simulink model "APPL_PaFaultDetection"  (R2018b)
settings: configuration reference "CodeConfig_10_ms" (kept outside this file)
undefined symbols (not defined in the file): CAL_LockErrNoTime_30ms, CAL_ManualSwValid_90s, CAL_MotorHallInvalid_2s, CAL_MotorMaxRunTime_60s, CAL_MotorRelayErr_2s, CAL_MotorStall_750ms, D_DrSoftStopDef_B, D_DrSoftStopDef_F, D_DrSoftStopDef_H, D_DrSoftStopDef_L, D_Relay_DownBackFault, D_Relay_UpFrontFault, D_StallCurrent, enSeatMoveCmd, FALSE, TRUE
libraries: DareLib x91, simulink x2
(part 2 of 4)

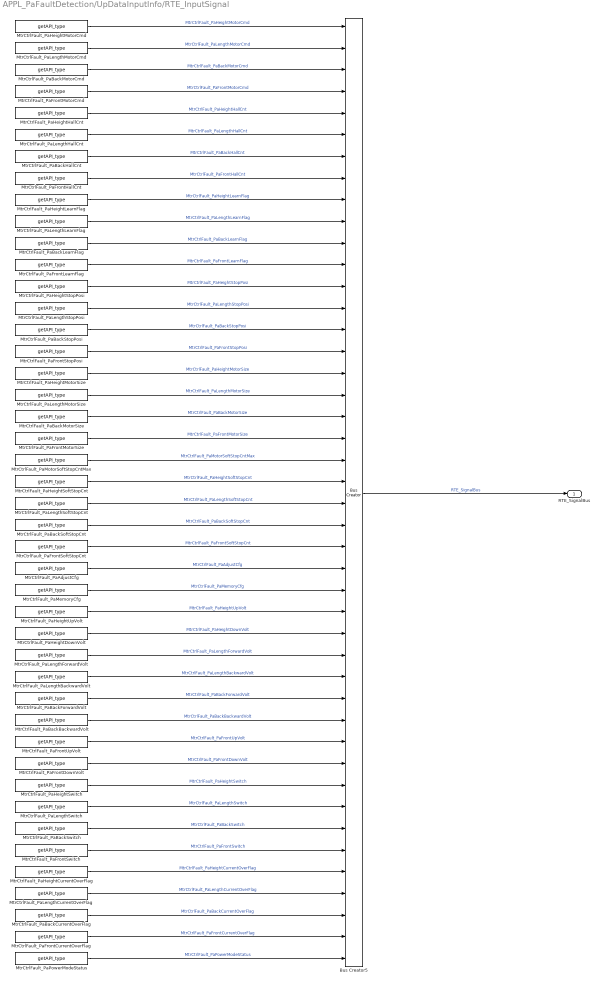
== system APPL_PaFaultDetection/UpDataInputInfo/RTE_InputSignal ==
  Bus Creator5 : BusCreator  Inputs=44
  MtrCtrlFault_PaAdjustCfg : DareLib/Dare/getAPI_type  g_funcname=Srvl_GetMemIndexDataU8  g_param=EN_MemIndex_PaAdjustConfig  g_type=uint8  g_size=-1
      settings: AttributesFormatString=%<g_funcname>  SourceProductName=Dare Library
  MtrCtrlFault_PaBackBackwardVolt : DareLib/Dare/getAPI_type  g_funcname=Ecual_GetPaRelayFlagBackBackward  g_param=""  g_type=uint8  g_size=-1
      settings: AttributesFormatString=%<g_funcname>  SourceProductName=Dare Library
  MtrCtrlFault_PaBackCurrentOverFlag : DareLib/Dare/getAPI_type  g_funcname=Ecual_GetPrBackOverCurrentFlag  g_param=""  g_type=uint8  g_size=-1
      settings: AttributesFormatString=%<g_funcname>  SourceProductName=Dare Library
  MtrCtrlFault_PaBackForwardVolt : DareLib/Dare/getAPI_type  g_funcname=Ecual_GetPaRelayFlagBackForward  g_param=""  g_type=uint8  g_size=-1
      settings: AttributesFormatString=%<g_funcname>  SourceProductName=Dare Library
  MtrCtrlFault_PaBackHallCnt : DareLib/Dare/getAPI_type  g_funcname=Cdd_GetCurrentHallCnt  g_param=EN_PassengerBack  g_type=uint16  g_size=-1
      settings: AttributesFormatString=%<g_funcname>  SourceProductName=Dare Library
  MtrCtrlFault_PaBackLearnFlag : DareLib/Dare/getAPI_type  g_funcname=Cdd_GetMotorLearnFlag  g_param=EN_PassengerBack  g_type=uint8  g_size=-1
      settings: AttributesFormatString=%<g_funcname>  SourceProductName=Dare Library
  MtrCtrlFault_PaBackMotorCmd : DareLib/Dare/getAPI_type  g_funcname=Rte_GetVfb_PaBackMotorCmd  g_param=""  g_type=uint8  g_size=-1
      settings: AttributesFormatString=%<g_funcname>  SourceProductName=Dare Library
  MtrCtrlFault_PaBackMotorSize : DareLib/Dare/getAPI_type  g_funcname=Cdd_GetMotorSize  g_param=EN_PassengerBack  g_type=uint16  g_size=-1
      settings: AttributesFormatString=%<g_funcname>  SourceProductName=Dare Library
  MtrCtrlFault_PaBackSoftStopCnt : DareLib/Dare/getAPI_type  g_funcname=Srvl_GetMemIndexDataU8  g_param=EN_MemIndex_PaBackSoftStopCnt  g_type=uint8  g_size=-1
      settings: AttributesFormatString=%<g_funcname>  SourceProductName=Dare Library
  MtrCtrlFault_PaBackStopPosi : DareLib/Dare/getAPI_type  g_funcname=Cdd_GetMotorHardStop  g_param=EN_PassengerBack  g_type=uint16  g_size=-1
      settings: AttributesFormatString=%<g_funcname>  SourceProductName=Dare Library
  MtrCtrlFault_PaBackSwitch : DareLib/Dare/getAPI_type  g_funcname=Ecual_GetPaBackSwitchCmd  g_param=""  g_type=uint8  g_enum=enSeatMoveCmd  g_size=-1
      settings: AttributesFormatString=%<g_funcname>  SourceProductName=Dare Library
  MtrCtrlFault_PaFrontCurrentOverFlag : DareLib/Dare/getAPI_type  g_funcname=Ecual_GetPrFrontOverCurrentFlag  g_param=""  g_type=uint8  g_size=-1
      settings: AttributesFormatString=%<g_funcname>  SourceProductName=Dare Library
  MtrCtrlFault_PaFrontDownVolt : DareLib/Dare/getAPI_type  g_funcname=Ecual_GetPaRelayFlagFrontDown  g_param=""  g_type=uint8  g_size=-1
      settings: AttributesFormatString=%<g_funcname>  SourceProductName=Dare Library
  MtrCtrlFault_PaFrontHallCnt : DareLib/Dare/getAPI_type  g_funcname=Cdd_GetCurrentHallCnt  g_param=EN_PaResever_2  g_type=uint16  g_size=-1
      settings: AttributesFormatString=%<g_funcname>  SourceProductName=Dare Library
  MtrCtrlFault_PaFrontLearnFlag : DareLib/Dare/getAPI_type  g_funcname=Cdd_GetMotorLearnFlag  g_param=EN_PaResever_2  g_type=uint8  g_size=-1
      settings: AttributesFormatString=%<g_funcname>  SourceProductName=Dare Library
  MtrCtrlFault_PaFrontMotorCmd : DareLib/Dare/getAPI_type  g_funcname=Rte_GetVfb_PaFrontMotorCmd  g_param=""  g_type=uint8  g_size=-1
      settings: AttributesFormatString=%<g_funcname>  SourceProductName=Dare Library
  MtrCtrlFault_PaFrontMotorSize : DareLib/Dare/getAPI_type  g_funcname=Cdd_GetMotorSize  g_param=EN_PaResever_2  g_type=uint16  g_size=-1
      settings: AttributesFormatString=%<g_funcname>  SourceProductName=Dare Library
  MtrCtrlFault_PaFrontSoftStopCnt : DareLib/Dare/getAPI_type  g_funcname=Srvl_GetMemIndexDataU8  g_param=EN_MemIndex_PaFrontSoftStopCnt  g_type=uint8  g_size=-1
      settings: AttributesFormatString=%<g_funcname>  SourceProductName=Dare Library
  MtrCtrlFault_PaFrontStopPosi : DareLib/Dare/getAPI_type  g_funcname=Cdd_GetMotorHardStop  g_param=EN_PaResever_2  g_type=uint16  g_size=-1
      settings: AttributesFormatString=%<g_funcname>  SourceProductName=Dare Library
  MtrCtrlFault_PaFrontSwitch : DareLib/Dare/getAPI_type  g_funcname=Ecual_GetPaFrontSwitchCmd  g_param=""  g_type=uint8  g_enum=enSeatMoveCmd  g_size=-1
      settings: AttributesFormatString=%<g_funcname>  SourceProductName=Dare Library
  MtrCtrlFault_PaFrontUpVolt : DareLib/Dare/getAPI_type  g_funcname=Ecual_GetPaRelayFlagFrontUp  g_param=""  g_type=uint8  g_size=-1
      settings: AttributesFormatString=%<g_funcname>  SourceProductName=Dare Library
  MtrCtrlFault_PaHeightCurrentOverFlag : DareLib/Dare/getAPI_type  g_funcname=Ecual_GetPrHeightOverCurrentFlag  g_param=""  g_type=uint8  g_size=-1
      settings: AttributesFormatString=%<g_funcname>  SourceProductName=Dare Library
  MtrCtrlFault_PaHeightDownVolt : DareLib/Dare/getAPI_type  g_funcname=Ecual_GetPaRelayFlagHeightDN  g_param=""  g_type=uint8  g_size=-1
      settings: AttributesFormatString=%<g_funcname>  SourceProductName=Dare Library
  MtrCtrlFault_PaHeightHallCnt : DareLib/Dare/getAPI_type  g_funcname=Cdd_GetCurrentHallCnt  g_param=EN_PaResever_1  g_type=uint16  g_size=-1
      settings: AttributesFormatString=%<g_funcname>  SourceProductName=Dare Library
  MtrCtrlFault_PaHeightLearnFlag : DareLib/Dare/getAPI_type  g_funcname=Cdd_GetMotorLearnFlag  g_param=EN_PaResever_1  g_type=uint8  g_size=-1
      settings: AttributesFormatString=%<g_funcname>  SourceProductName=Dare Library
  MtrCtrlFault_PaHeightMotorCmd : DareLib/Dare/getAPI_type  g_funcname=Rte_GetVfb_PaHeightMotorCmd  g_param=""  g_type=uint8  g_size=-1
      settings: AttributesFormatString=%<g_funcname>  SourceProductName=Dare Library
  MtrCtrlFault_PaHeightMotorSize : DareLib/Dare/getAPI_type  g_funcname=Cdd_GetMotorSize  g_param=EN_PaResever_1  g_type=uint16  g_size=-1
      settings: AttributesFormatString=%<g_funcname>  SourceProductName=Dare Library
  MtrCtrlFault_PaHeightSoftStopCnt : DareLib/Dare/getAPI_type  g_funcname=Srvl_GetMemIndexDataU8  g_param=EN_MemIndex_PaHeightSoftStopCnt  g_type=uint8  g_size=-1
      settings: AttributesFormatString=%<g_funcname>  SourceProductName=Dare Library
  MtrCtrlFault_PaHeightStopPosi : DareLib/Dare/getAPI_type  g_funcname=Cdd_GetMotorHardStop  g_param=EN_PaResever_1  g_type=uint16  g_size=-1
      settings: AttributesFormatString=%<g_funcname>  SourceProductName=Dare Library
  MtrCtrlFault_PaHeightSwitch : DareLib/Dare/getAPI_type  g_funcname=Ecual_GetPaHeightSwitchCmd  g_param=""  g_type=uint8  g_enum=enSeatMoveCmd  g_size=-1
      settings: AttributesFormatString=%<g_funcname>  SourceProductName=Dare Library
  MtrCtrlFault_PaHeightUpVolt : DareLib/Dare/getAPI_type  g_funcname=Ecual_GetPaRelayFlagHeightUp  g_param=""  g_type=uint8  g_size=-1
      settings: AttributesFormatString=%<g_funcname>  SourceProductName=Dare Library
  MtrCtrlFault_PaLengthBackwardVolt : DareLib/Dare/getAPI_type  g_funcname=Ecual_GetPaRelayFlagLenghtBackward  g_param=""  g_type=uint8  g_size=-1
      settings: AttributesFormatString=%<g_funcname>  SourceProductName=Dare Library
  MtrCtrlFault_PaLengthCurrentOverFlag : DareLib/Dare/getAPI_type  g_funcname=Ecual_GetPrLengthOverCurrentFlag  g_param=""  g_type=uint8  g_size=-1
      settings: AttributesFormatString=%<g_funcname>  SourceProductName=Dare Library
  MtrCtrlFault_PaLengthForwardVolt : DareLib/Dare/getAPI_type  g_funcname=Ecual_GetPaRelayFlagLenghtForward  g_param=""  g_type=uint8  g_size=-1
      settings: AttributesFormatString=%<g_funcname>  SourceProductName=Dare Library
  MtrCtrlFault_PaLengthHallCnt : DareLib/Dare/getAPI_type  g_funcname=Cdd_GetCurrentHallCnt  g_param=EN_PassengerLength  g_type=uint16  g_size=-1
      settings: AttributesFormatString=%<g_funcname>  SourceProductName=Dare Library
  MtrCtrlFault_PaLengthLearnFlag : DareLib/Dare/getAPI_type  g_funcname=Cdd_GetMotorLearnFlag  g_param=EN_PassengerLength  g_type=uint8  g_size=-1
      settings: AttributesFormatString=%<g_funcname>  SourceProductName=Dare Library
  MtrCtrlFault_PaLengthMotorCmd : DareLib/Dare/getAPI_type  g_funcname=Rte_GetVfb_PaLengthMotorCmd  g_param=""  g_type=uint8  g_size=-1
      settings: AttributesFormatString=%<g_funcname>  SourceProductName=Dare Library
  MtrCtrlFault_PaLengthMotorSize : DareLib/Dare/getAPI_type  g_funcname=Cdd_GetMotorSize  g_param=EN_PassengerLength  g_type=uint16  g_size=-1
      settings: AttributesFormatString=%<g_funcname>  SourceProductName=Dare Library
  MtrCtrlFault_PaLengthSoftStopCnt : DareLib/Dare/getAPI_type  g_funcname=Srvl_GetMemIndexDataU8  g_param=EN_MemIndex_PaLengthSoftStopCnt  g_type=uint8  g_size=-1
      settings: AttributesFormatString=%<g_funcname>  SourceProductName=Dare Library
  MtrCtrlFault_PaLengthStopPosi : DareLib/Dare/getAPI_type  g_funcname=Cdd_GetMotorHardStop  g_param=EN_PassengerLength  g_type=uint16  g_size=-1
      settings: AttributesFormatString=%<g_funcname>  SourceProductName=Dare Library
  MtrCtrlFault_PaLengthSwitch : DareLib/Dare/getAPI_type  g_funcname=Ecual_GetPaLengthSwitchCmd  g_param=""  g_type=uint8  g_enum=enSeatMoveCmd  g_size=-1
      settings: AttributesFormatString=%<g_funcname>  SourceProductName=Dare Library
  MtrCtrlFault_PaMemoryCfg : DareLib/Dare/getAPI_type  g_funcname=Srvl_GetMemIndexDataU8  g_param=EN_MemIndex_PaMemoryConfig  g_type=uint8  g_size=-1
      settings: AttributesFormatString=%<g_funcname>  SourceProductName=Dare Library
  MtrCtrlFault_PaMotorSoftStopCntMax : DareLib/Dare/getAPI_type  g_funcname=Srvl_GetMemIndexDataU8  g_param=EN_MemIndex_MotorSoftStopCntMax  g_type=uint8  g_size=-1
      settings: AttributesFormatString=%<g_funcname>  SourceProductName=Dare Library
  MtrCtrlFault_PaPowerModeStatus : DareLib/Dare/getAPI_type  g_funcname=Rte_GetVfb_PowerMode  g_param=""  g_type=uint8  g_enum=enIgnSts  g_size=-1
      settings: AttributesFormatString=%<g_funcname>  SourceProductName=Dare Library
  RTE_SignalBus : Outport
  wires:
  Bus Creator5/1 -> RTE_SignalBus/1  "RTE_SignalBus"
  MtrCtrlFault_PaHeightMotorCmd/1 -> Bus Creator5/1  "MtrCtrlFault_PaHeightMotorCmd"
  MtrCtrlFault_PaLengthMotorCmd/1 -> Bus Creator5/2  "MtrCtrlFault_PaLengthMotorCmd"
  MtrCtrlFault_PaBackMotorCmd/1 -> Bus Creator5/3  "MtrCtrlFault_PaBackMotorCmd"
  MtrCtrlFault_PaFrontMotorCmd/1 -> Bus Creator5/4  "MtrCtrlFault_PaFrontMotorCmd"
  MtrCtrlFault_PaHeightHallCnt/1 -> Bus Creator5/5  "MtrCtrlFault_PaHeightHallCnt"
  MtrCtrlFault_PaLengthHallCnt/1 -> Bus Creator5/6  "MtrCtrlFault_PaLengthHallCnt"
  MtrCtrlFault_PaBackHallCnt/1 -> Bus Creator5/7  "MtrCtrlFault_PaBackHallCnt"
  MtrCtrlFault_PaFrontHallCnt/1 -> Bus Creator5/8  "MtrCtrlFault_PaFrontHallCnt"
  MtrCtrlFault_PaHeightLearnFlag/1 -> Bus Creator5/9  "MtrCtrlFault_PaHeightLearnFlag"
  MtrCtrlFault_PaLengthLearnFlag/1 -> Bus Creator5/10  "MtrCtrlFault_PaLengthLearnFlag"
  MtrCtrlFault_PaBackLearnFlag/1 -> Bus Creator5/11  "MtrCtrlFault_PaBackLearnFlag"
  MtrCtrlFault_PaFrontLearnFlag/1 -> Bus Creator5/12  "MtrCtrlFault_PaFrontLearnFlag"
  MtrCtrlFault_PaHeightStopPosi/1 -> Bus Creator5/13  "MtrCtrlFault_PaHeightStopPosi"
  MtrCtrlFault_PaLengthStopPosi/1 -> Bus Creator5/14  "MtrCtrlFault_PaLengthStopPosi"
  MtrCtrlFault_PaBackStopPosi/1 -> Bus Creator5/15  "MtrCtrlFault_PaBackStopPosi"
  MtrCtrlFault_PaFrontStopPosi/1 -> Bus Creator5/16  "MtrCtrlFault_PaFrontStopPosi"
  MtrCtrlFault_PaHeightMotorSize/1 -> Bus Creator5/17  "MtrCtrlFault_PaHeightMotorSize"
  MtrCtrlFault_PaLengthMotorSize/1 -> Bus Creator5/18  "MtrCtrlFault_PaLengthMotorSize"
  MtrCtrlFault_PaBackMotorSize/1 -> Bus Creator5/19  "MtrCtrlFault_PaBackMotorSize"
  MtrCtrlFault_PaFrontMotorSize/1 -> Bus Creator5/20  "MtrCtrlFault_PaFrontMotorSize"
  MtrCtrlFault_PaMotorSoftStopCntMax/1 -> Bus Creator5/21  "MtrCtrlFault_PaMotorSoftStopCntMax"
  MtrCtrlFault_PaHeightSoftStopCnt/1 -> Bus Creator5/22  "MtrCtrlFault_PaHeightSoftStopCnt"
  MtrCtrlFault_PaLengthSoftStopCnt/1 -> Bus Creator5/23  "MtrCtrlFault_PaLengthSoftStopCnt"
  MtrCtrlFault_PaBackSoftStopCnt/1 -> Bus Creator5/24  "MtrCtrlFault_PaBackSoftStopCnt"
  MtrCtrlFault_PaFrontSoftStopCnt/1 -> Bus Creator5/25  "MtrCtrlFault_PaFrontSoftStopCnt"
  MtrCtrlFault_PaAdjustCfg/1 -> Bus Creator5/26  "MtrCtrlFault_PaAdjustCfg"
  MtrCtrlFault_PaMemoryCfg/1 -> Bus Creator5/27  "MtrCtrlFault_PaMemoryCfg"
  MtrCtrlFault_PaHeightUpVolt/1 -> Bus Creator5/28  "MtrCtrlFault_PaHeightUpVolt"
  MtrCtrlFault_PaHeightDownVolt/1 -> Bus Creator5/29  "MtrCtrlFault_PaHeightDownVolt"
  MtrCtrlFault_PaLengthForwardVolt/1 -> Bus Creator5/30  "MtrCtrlFault_PaLengthForwardVolt"
  MtrCtrlFault_PaLengthBackwardVolt/1 -> Bus Creator5/31  "MtrCtrlFault_PaLengthBackwardVolt"
  MtrCtrlFault_PaBackForwardVolt/1 -> Bus Creator5/32  "MtrCtrlFault_PaBackForwardVolt"
  MtrCtrlFault_PaBackBackwardVolt/1 -> Bus Creator5/33  "MtrCtrlFault_PaBackBackwardVolt"
  MtrCtrlFault_PaFrontUpVolt/1 -> Bus Creator5/34  "MtrCtrlFault_PaFrontUpVolt"
  MtrCtrlFault_PaFrontDownVolt/1 -> Bus Creator5/35  "MtrCtrlFault_PaFrontDownVolt"
  MtrCtrlFault_PaHeightSwitch/1 -> Bus Creator5/36  "MtrCtrlFault_PaHeightSwitch"
  MtrCtrlFault_PaLengthSwitch/1 -> Bus Creator5/37  "MtrCtrlFault_PaLengthSwitch"
  MtrCtrlFault_PaBackSwitch/1 -> Bus Creator5/38  "MtrCtrlFault_PaBackSwitch"
  MtrCtrlFault_PaFrontSwitch/1 -> Bus Creator5/39  "MtrCtrlFault_PaFrontSwitch"
  MtrCtrlFault_PaHeightCurrentOverFlag/1 -> Bus Creator5/40  "MtrCtrlFault_PaHeightCurrentOverFlag"
  MtrCtrlFault_PaLengthCurrentOverFlag/1 -> Bus Creator5/41  "MtrCtrlFault_PaLengthCurrentOverFlag"
  MtrCtrlFault_PaBackCurrentOverFlag/1 -> Bus Creator5/42  "MtrCtrlFault_PaBackCurrentOverFlag"
  MtrCtrlFault_PaFrontCurrentOverFlag/1 -> Bus Creator5/43  "MtrCtrlFault_PaFrontCurrentOverFlag"
  MtrCtrlFault_PaPowerModeStatus/1 -> Bus Creator5/44  "MtrCtrlFault_PaPowerModeStatus"

== system APPL_PaFaultDetection/LogicCtrl/AdheAndEffec/SwitchErrorDetection/GetCurMsTs ==
  f : TriggerPort  TriggerType=function-call  VariantControl=(inherit)
      settings: CopyFcn=Stateflow.SLINSF.SimulinkMan.removeBlockPreDeleteFcn  PreDeleteFcn=Stateflow.SLINSF.SimulinkMan.unsafePredeleteFcn
  DrAdj_LenAdjSize : DareLib/Dare/getAPI_type  g_funcname=D_HAL_GET_CUR_MS_TS  g_param=""  g_type=uint32  g_size=-1
      settings: SourceProductName=Dare Library
  Ts : Outport
  wires:
  DrAdj_LenAdjSize/1 -> Ts/1  "DrAdj_CurMsTs"

== system APPL_PaFaultDetection/LogicCtrl/AdheAndEffec/SwitchErrorDetection/GetDefTime ==
  DefTs : Inport
  Ts : Inport  Port=2
  f : TriggerPort  TriggerType=function-call  VariantControl=(inherit)
      settings: CopyFcn=Stateflow.SLINSF.SimulinkMan.removeBlockPreDeleteFcn  PreDeleteFcn=Stateflow.SLINSF.SimulinkMan.unsafePredeleteFcn
  Chart : Stateflow chart  TreatAsAtomicUnit=on
  OutTs : Outport
  wires:
  DefTs/1 -> Chart/1(DefTs)
  Ts/1 -> Chart/2(Ts)
  Chart/1(OutTs) -> OutTs/1

== system APPL_PaFaultDetection/LogicCtrl/AdheAndEffec/SwitchErrorDetection/TimeDiffTs ==
  lastTs : Inport
  Ts : Inport  Port=2
  f : TriggerPort  TriggerType=function-call  VariantControl=(inherit)
      settings: CopyFcn=Stateflow.SLINSF.SimulinkMan.removeBlockPreDeleteFcn  PreDeleteFcn=Stateflow.SLINSF.SimulinkMan.unsafePredeleteFcn
  Chart : Stateflow chart  TreatAsAtomicUnit=on
  OutTs : Outport
  wires:
  lastTs/1 -> Chart/1(lastTs)
  Ts/1 -> Chart/2(Ts)
  Chart/1(OutTs) -> OutTs/1

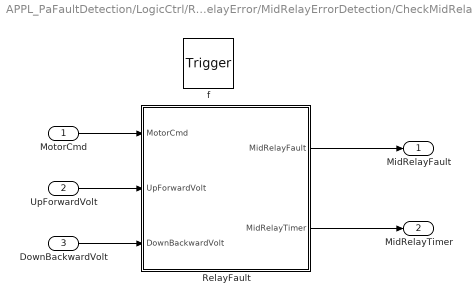
== system APPL_PaFaultDetection/LogicCtrl/RelayError/MidRelayErrorDetection/CheckMidRelayFault ==
  MotorCmd : Inport  OutDataTypeStr=uint8  PortDimensions=1
  UpForwardVolt : Inport  Port=2  OutDataTypeStr=uint8  PortDimensions=1
  DownBackwardVolt : Inport  Port=3  OutDataTypeStr=uint8  PortDimensions=1
  f : TriggerPort  TriggerType=function-call  VariantControl=(inherit)
      settings: CopyFcn=Stateflow.SLINSF.SimulinkMan.removeBlockPreDeleteFcn  PreDeleteFcn=Stateflow.SLINSF.SimulinkMan.unsafePredeleteFcn
  RelayFault : Stateflow chart  TreatAsAtomicUnit=on
  MidRelayFault : Outport  OutDataTypeStr=uint8
  MidRelayTimer : Outport  Port=2  OutDataTypeStr=uint8
  wires:
  MotorCmd/1 -> RelayFault/1(MotorCmd)
  UpForwardVolt/1 -> RelayFault/2(UpForwardVolt)
  DownBackwardVolt/1 -> RelayFault/3(DownBackwardVolt)
  RelayFault/1(MidRelayFault) -> MidRelayFault/1
  RelayFault/2(MidRelayTimer) -> MidRelayTimer/1

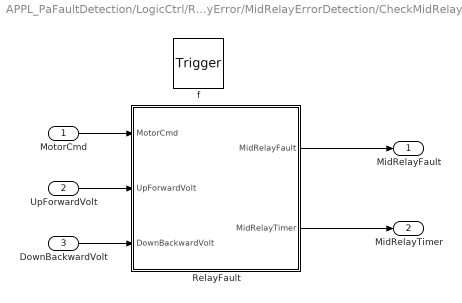
== system APPL_PaFaultDetection/LogicCtrl/RelayError/MidRelayErrorDetection/CheckMidRelayFault1 ==
  MotorCmd : Inport  OutDataTypeStr=uint8  PortDimensions=1
  UpForwardVolt : Inport  Port=2  OutDataTypeStr=uint8  PortDimensions=1
  DownBackwardVolt : Inport  Port=3  OutDataTypeStr=uint8  PortDimensions=1
  f : TriggerPort  TriggerType=function-call  VariantControl=(inherit)
      settings: CopyFcn=Stateflow.SLINSF.SimulinkMan.removeBlockPreDeleteFcn  PreDeleteFcn=Stateflow.SLINSF.SimulinkMan.unsafePredeleteFcn
  RelayFault : Stateflow chart  TreatAsAtomicUnit=on
  MidRelayFault : Outport  OutDataTypeStr=uint8
  MidRelayTimer : Outport  Port=2  OutDataTypeStr=uint8
  wires:
  MotorCmd/1 -> RelayFault/1(MotorCmd)
  UpForwardVolt/1 -> RelayFault/2(UpForwardVolt)
  DownBackwardVolt/1 -> RelayFault/3(DownBackwardVolt)
  RelayFault/1(MidRelayFault) -> MidRelayFault/1
  RelayFault/2(MidRelayTimer) -> MidRelayTimer/1

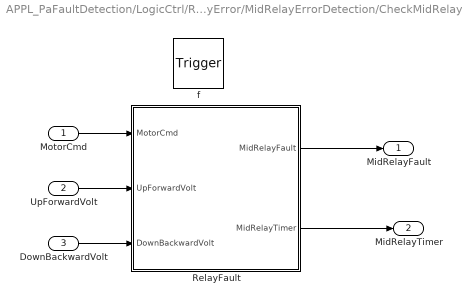
== system APPL_PaFaultDetection/LogicCtrl/RelayError/MidRelayErrorDetection/CheckMidRelayFault2 ==
  MotorCmd : Inport  OutDataTypeStr=uint8  PortDimensions=1
  UpForwardVolt : Inport  Port=2  OutDataTypeStr=uint8  PortDimensions=1
  DownBackwardVolt : Inport  Port=3  OutDataTypeStr=uint8  PortDimensions=1
  f : TriggerPort  TriggerType=function-call  VariantControl=(inherit)
      settings: CopyFcn=Stateflow.SLINSF.SimulinkMan.removeBlockPreDeleteFcn  PreDeleteFcn=Stateflow.SLINSF.SimulinkMan.unsafePredeleteFcn
  RelayFault : Stateflow chart  TreatAsAtomicUnit=on
  MidRelayFault : Outport  OutDataTypeStr=uint8
  MidRelayTimer : Outport  Port=2  OutDataTypeStr=uint8
  wires:
  MotorCmd/1 -> RelayFault/1(MotorCmd)
  UpForwardVolt/1 -> RelayFault/2(UpForwardVolt)
  DownBackwardVolt/1 -> RelayFault/3(DownBackwardVolt)
  RelayFault/1(MidRelayFault) -> MidRelayFault/1
  RelayFault/2(MidRelayTimer) -> MidRelayTimer/1

== system APPL_PaFaultDetection/LogicCtrl/RelayError/MidRelayErrorDetection/CheckMidRelayFault3 ==
  MotorCmd : Inport  OutDataTypeStr=uint8  PortDimensions=1
  UpForwardVolt : Inport  Port=2  OutDataTypeStr=uint8  PortDimensions=1
  DownBackwardVolt : Inport  Port=3  OutDataTypeStr=uint8  PortDimensions=1
  f : TriggerPort  TriggerType=function-call  VariantControl=(inherit)
      settings: CopyFcn=Stateflow.SLINSF.SimulinkMan.removeBlockPreDeleteFcn  PreDeleteFcn=Stateflow.SLINSF.SimulinkMan.unsafePredeleteFcn
  RelayFault : Stateflow chart  TreatAsAtomicUnit=on
  MidRelayFault : Outport  OutDataTypeStr=uint8
  MidRelayTimer : Outport  Port=2  OutDataTypeStr=uint8
  wires:
  MotorCmd/1 -> RelayFault/1(MotorCmd)
  UpForwardVolt/1 -> RelayFault/2(UpForwardVolt)
  DownBackwardVolt/1 -> RelayFault/3(DownBackwardVolt)
  RelayFault/1(MidRelayFault) -> MidRelayFault/1
  RelayFault/2(MidRelayTimer) -> MidRelayTimer/1

== system APPL_PaFaultDetection/LogicCtrl/SoftStopPoint/SoftStopPointDetection/DrAdj_SetBackSoftStopCnt ==
  Cnt : Inport
  f : TriggerPort  TriggerType=function-call  VariantControl=(inherit)
      settings: CopyFcn=Stateflow.SLINSF.SimulinkMan.removeBlockPreDeleteFcn  PreDeleteFcn=Stateflow.SLINSF.SimulinkMan.unsafePredeleteFcn
  DriverFrontMoveType12 : DareLib/Dare/setAPI_type  g_funcname=Srvl_SetMemIndexDataU8  g_param=EN_MemIndex_PaBackSoftStopCnt  g_type=uint8  g_size=-1
      settings: AttributesFormatString=%<g_funcname>  SourceProductName=Dare Library
  wires:
  Cnt/1 -> DriverFrontMoveType12/1

== system APPL_PaFaultDetection/LogicCtrl/SoftStopPoint/SoftStopPointDetection/DrAdj_SetFrontSoftStopCnt ==
  Cnt : Inport
  f : TriggerPort  TriggerType=function-call  VariantControl=(inherit)
      settings: CopyFcn=Stateflow.SLINSF.SimulinkMan.removeBlockPreDeleteFcn  PreDeleteFcn=Stateflow.SLINSF.SimulinkMan.unsafePredeleteFcn
  DriverFrontMoveType12 : DareLib/Dare/setAPI_type  g_funcname=Srvl_SetMemIndexDataU8  g_param=EN_MemIndex_PaFrontSoftStopCnt  g_type=uint8  g_size=-1
      settings: AttributesFormatString=%<g_funcname>  SourceProductName=Dare Library
  wires:
  Cnt/1 -> DriverFrontMoveType12/1

== system APPL_PaFaultDetection/LogicCtrl/SoftStopPoint/SoftStopPointDetection/DrAdj_SetHeightSoftStopCnt ==
  Cnt : Inport
  f : TriggerPort  TriggerType=function-call  VariantControl=(inherit)
      settings: CopyFcn=Stateflow.SLINSF.SimulinkMan.removeBlockPreDeleteFcn  PreDeleteFcn=Stateflow.SLINSF.SimulinkMan.unsafePredeleteFcn
  DriverFrontMoveType12 : DareLib/Dare/setAPI_type  g_funcname=Srvl_SetMemIndexDataU8  g_param=EN_MemIndex_PaHeightSoftStopCnt  g_type=uint8  g_size=-1
      settings: AttributesFormatString=%<g_funcname>  SourceProductName=Dare Library
  wires:
  Cnt/1 -> DriverFrontMoveType12/1

== system APPL_PaFaultDetection/LogicCtrl/SoftStopPoint/SoftStopPointDetection/DrAdj_SetLengthSoftStopCnt ==
  Cnt : Inport
  f : TriggerPort  TriggerType=function-call  VariantControl=(inherit)
      settings: CopyFcn=Stateflow.SLINSF.SimulinkMan.removeBlockPreDeleteFcn  PreDeleteFcn=Stateflow.SLINSF.SimulinkMan.unsafePredeleteFcn
  DriverFrontMoveType12 : DareLib/Dare/setAPI_type  g_funcname=Srvl_SetMemIndexDataU8  g_param=EN_MemIndex_PaLengthSoftStopCnt  g_type=uint8  g_size=-1
      settings: AttributesFormatString=%<g_funcname>  SourceProductName=Dare Library
  wires:
  Cnt/1 -> DriverFrontMoveType12/1

== stateflow chart APPL_PaFaultDetection/LogicCtrl/SwitchErrDeal/ SWProcess  ==
  settings: description=硬线开关信号处理 SWProcess
  state DSM_SWAdjust
    state HeightSWProcess [parallel] [commented out]
      state Enable [commented out]
        en:
        CurrentHeightSwCmd =DrMtr_HeightSwitchCmd;
        du:
        CurrentHeightSwCmd =DrMtr_HeightSwitchCmd;
      state Disable [commented out]
        en:
        CurrentHeightSwCmd = FALSE;
      (default) -> DSM_SWAdjust.HeightSWProcess.Disable [commented out]
      DSM_SWAdjust.HeightSWProcess.Disable -> DSM_SWAdjust.HeightSWProcess.Enable [commented out] : /* 高度本地开关命令故障处理 */
          | [DrMtr_HeightSwitchCmd !=FALSE ...
          | &&FALSE == DrMtr_HeightSwitchAdheErr ...
          | && FALSE ==DrMtr_HeightRelayAdhesionErr ...
          | &&FALSE == DrMtr_HeightStallErr]
      DSM_SWAdjust.HeightSWProcess.Enable -> DSM_SWAdjust.HeightSWProcess.Disable [commented out] : [DrMtr_HeightSwitchCmd ==FALSE ...
          | || FALSE != DrMtr_HeightSwitchAdheErr ...
          | || TRUE == DrMtr_HeightRelayAdhesionErr ...
          | || TRUE == DrMtr_HeightStallErr]
    state LengthSWProcess [parallel]
      settings: executionOrder=1
      state Enable
        en:
        CurrentLengthSwCmd =DrMtr_LengthSwitchCmd;
        du:
        CurrentLengthSwCmd =DrMtr_LengthSwitchCmd;
      state Disable
        en:
        CurrentLengthSwCmd = FALSE;
      (default) -> DSM_SWAdjust.LengthSWProcess.Disable
      DSM_SWAdjust.LengthSWProcess.Disable -> DSM_SWAdjust.LengthSWProcess.Enable : /* 纵向本地开关命令故障处理 */
          | [DrMtr_LengthSwitchCmd !=FALSE ...
          | &&FALSE == DrMtr_LengthSwitchAdheErr...
          | && FALSE ==DrMtr_LengthRelayAdhesionErr ...
          | &&FALSE == DrMtr_LengthStallErr]
      DSM_SWAdjust.LengthSWProcess.Enable -> DSM_SWAdjust.LengthSWProcess.Disable : [DrMtr_LengthSwitchCmd ==FALSE ...
          | || FALSE !=  DrMtr_LengthSwitchAdheErr...
          | || TRUE == DrMtr_LengthRelayAdhesionErr ...
          | || TRUE == DrMtr_LengthStallErr]
    state BackSWProcess [parallel]
      settings: executionOrder=2
      state Enable
        en:
        CurrentBackSwCmd =DrMtr_BackSwitchCmd;
        du:
        CurrentBackSwCmd =DrMtr_BackSwitchCmd;
      state Disable
        en:
        CurrentBackSwCmd = FALSE;
      (default) -> DSM_SWAdjust.BackSWProcess.Disable
      DSM_SWAdjust.BackSWProcess.Disable -> DSM_SWAdjust.BackSWProcess.Enable : /* 靠背本地开关命令故障处理 */
          | [DrMtr_BackSwitchCmd !=FALSE ...
          | &&FALSE == DrMtr_BackRelayAdhesionErr ...
          | &&FALSE == DrMtr_BackSwitchAdheErr...
          | &&FALSE == DrMtr_BackStallErr]
      DSM_SWAdjust.BackSWProcess.Enable -> DSM_SWAdjust.BackSWProcess.Disable : [DrMtr_BackSwitchCmd ==FALSE ...
          | || FALSE != DrMtr_BackRelayAdhesionErr ...
          | || TRUE == DrMtr_BackSwitchAdheErr...
          | || TRUE == DrMtr_BackStallErr]
    state FrontSWProcess [parallel] [commented out]
      state Enable [commented out]
        en:
        CurrentFrontSwCmd =DrMtr_FrontSwitchCmd;
        du:
        CurrentFrontSwCmd =DrMtr_FrontSwitchCmd;
      state Disable [commented out]
        en:
        CurrentFrontSwCmd = FALSE;
      (default) -> DSM_SWAdjust.FrontSWProcess.Disable [commented out]
      DSM_SWAdjust.FrontSWProcess.Disable -> DSM_SWAdjust.FrontSWProcess.Enable [commented out] : /* 腿托本地开关命令故障处理 && 配置字满足*/
          | [DrMtr_FrontSwitchCmd !=FALSE ...
          | && FALSE == DrMtr_FrontSwitchAdheErr...
          | && FALSE ==DrMtr_FrontRelayAdhesionErr ...
          | && FALSE == DrMtr_FrontStallErr ...
          | && EN_DrTwelveWayMotor == MtrCtrlFault_DrAdjustCfg]
      DSM_SWAdjust.FrontSWProcess.Enable -> DSM_SWAdjust.FrontSWProcess.Disable [commented out] : [DrMtr_FrontSwitchCmd ==FALSE ...
          | || FALSE !=  DrMtr_FrontSwitchAdheErr...
          | || TRUE == DrMtr_FrontRelayAdhesionErr ...
          | || TRUE == DrMtr_FrontStallErr...
          | || EN_DrTwelveWayMotor != MtrCtrlFault_DrAdjustCfg]
  state Init
    en:
    CurrentHeightSwCmd = FALSE;
    CurrentLengthSwCmd = FALSE;
    CurrentBackSwCmd = FALSE;
    CurrentFrontSwCmd = FALSE;
  (default) -> Init
  Init -> DSM_SWAdjust : /* 非CRANK档位 且非不可调节配置 */
      | [eCrank != MtrCtrlFault_PowerModeStatus ...
      | && TRUE == MtrCtrlFault_DrAdjustCfg]
  DSM_SWAdjust -> Init : /* crank档 或 不可调节配置 */
      | [eCrank == MtrCtrlFault_PowerModeStatus ...
      | || TRUE != MtrCtrlFault_DrAdjustCfg]
  data: CurrentHeightSwCmd output Enum: enSeatMoveCmd; CurrentLengthSwCmd output Enum: enSeatMoveCmd; CurrentBackSwCmd output Enum: enSeatMoveCmd; DrMtr_HeightSwitchCmd input; DrMtr_LengthSwitchCmd input; DrMtr_BackSwitchCmd input; DrMtr_FrontSwitchCmd input; DrMtr_HeightRelayAdhesionErr input; DrMtr_LengthRelayAdhesionErr input; DrMtr_BackRelayAdhesionErr input; DrMtr_FrontRelayAdhesionErr input; DrMtr_HeightSwitchAdheErr input; DrMtr_LengthSwitchAdheErr input; DrMtr_BackSwitchAdheErr input; DrMtr_FrontSwitchAdheErr input; CurrentFrontSwCmd output Enum: enSeatMoveCmd; FALSE parameter; TRUE parameter; DrMtr_HeightStallErr input; DrMtr_LengthStallErr input; DrMtr_BackStallErr input; DrMtr_FrontStallErr input; MtrCtrlFault_DrAdjustCfg input; MtrCtrlFault_PowerModeStatus input

== stateflow chart APPL_PaFaultDetection/LogicCtrl/RelayError/MidRelayErrorDetection ==
  state [MidRelayFault,MidRelayTimer]  = CheckMidRelayFault(MotorCmd,UpForwardVolt,DownBackwardVolt) [function]
  state [MidRelayFault,MidRelayTimer] = CheckMidRelayFault1(MotorCmd,UpForwardVolt,DownBackwardVolt) [function]
  state [MidRelayFault,MidRelayTimer]  = CheckMidRelayFault2(MotorCmd,UpForwardVolt,DownBackwardVolt) [function]
  state [MidRelayFault,MidRelayTimer]  = CheckMidRelayFault3(MotorCmd,UpForwardVolt,DownBackwardVolt) [function]
  state MidRelayError [parallel]
    settings: executionOrder=1
    (default) -> (junction 66)
    MidRelayError -> (junction 66)
    (junction 66) -> (junction 68) : {/*[HeightMidRelayFault, HeightMidRelayTimer] = CheckMidRelayFault(MtrCtrlFault_HeightMotorCmd,MtrCtrlFault_HeightUpVolt,MtrCtrlFault_HeightDownVolt);*/
        | [LengthMidRelayFault, LengthMidRelayTimer] = CheckMidRelayFault1(MtrCtrlFault_LengthMotorCmd,MtrCtrlFault_LengthForwardVolt,MtrCtrlFault_LengthBackwardVolt);
        | [BackMidRelayFault, BackMidRelayTimer] = CheckMidRelayFault2(MtrCtrlFault_BackMotorCmd,MtrCtrlFault_BackForwardVolt,MtrCtrlFault_BackBackwardVolt);
        | /*[FrontMidRelayFault, FrontMidRelayTimer] = CheckMidRelayFault3(MtrCtrlFault_FrontMotorCmd,MtrCtrlFault_FrontUpVolt,MtrCtrlFault_FrontDownVolt);*/}
  note: 继电器粘连故障检测
  data: MotorCmd function_input uint8 size=1; UpForwardVolt function_input uint8 size=1; DownBackwardVolt function_input uint8 size=1; MidRelayFault function_output uint8; MidRelayTimer function_output uint8; MotorCmd function_input uint8 size=1; UpForwardVolt function_input uint8 size=1; DownBackwardVolt function_input uint8 size=1; MidRelayFault function_output uint8; MidRelayTimer function_output uint8; MotorCmd function_input uint8 size=1; UpForwardVolt function_input uint8 size=1; DownBackwardVolt function_input uint8 size=1; MidRelayFault function_output uint8; MidRelayTimer function_output uint8; MotorCmd function_input uint8 size=1; UpForwardVolt function_input uint8 size=1; DownBackwardVolt function_input uint8 size=1; MidRelayFault function_output uint8; MidRelayTimer function_output uint8; MtrCtrlFault_HeightUpVolt input uint8; MtrCtrlFault_HeightDownVolt input uint8; MtrCtrlFault_LengthForwardVolt input uint8; MtrCtrlFault_LengthBackwardVolt input uint8; MtrCtrlFault_BackForwardVolt input uint8; MtrCtrlFault_BackBackwardVolt input uint8; MtrCtrlFault_FrontUpVolt input uint8; MtrCtrlFault_FrontDownVolt input uint8; MtrCtrlFault_HeightMotorCmd input uint8; MtrCtrlFault_LengthMotorCmd input uint8; MtrCtrlFault_BackMotorCmd input uint8; MtrCtrlFault_FrontMotorCmd input uint8; HeightMidRelayFault output uint8; LengthMidRelayFault output uint8; BackMidRelayFault output uint8; FrontMidRelayFault output uint8; LengthMidRelayTimer local double; BackMidRelayTimer local double; FrontMidRelayTimer local double; HeightMidRelayTimer local double

== stateflow chart APPL_PaFaultDetection/LogicCtrl/RelayError/MidRelayErrorDetection/CheckMidRelayFault/RelayFault ==
  state Judge
    ex:
    MidRelayTimer = 0;
    (default) -> (junction 8)
    Judge -> (junction 8) [order 1]
    (junction 8) -> (junction 10) [order 1] : [CAL_MotorRelayErr_2s <= MidRelayTimer]
    (junction 8) -> (junction 14) [order 2] : {MidRelayTimer ++;}
    (junction 10) -> (junction 12) : {MidRelayTimer = CAL_MotorRelayErr_2s;}
    (junction 12) -> (junction 16) [order 1] : [enSeatMoveCmd.EN_UP_FORWARD != MotorCmd ...
        | && FALSE != UpForwardVolt]
    (junction 12) -> (junction 20) [order 2]
    (junction 16) -> (junction 18) : {MidRelayFault = D_Relay_UpFrontFault;}
    (junction 20) -> (junction 23) [order 1] : [enSeatMoveCmd.EN_DN_BACKWARD != MotorCmd ...
        | && FALSE != DownBackwardVolt]
    (junction 20) -> (junction 27) [order 2]
    (junction 23) -> (junction 25) : {MidRelayFault = D_Relay_DownBackFault;}
    (junction 14) -> (junction 27)
    (junction 25) -> (junction 27)
    (junction 18) -> (junction 25)
    (junction 27) -> (junction 31)
  state Normal
    en:
    MidRelayFault = FALSE;
    MidRelayTimer = 0;
  (default) -> Normal
  Normal -> Judge [order 1] : [/*没有输出命令但输出反馈有电压 满足前置条件*/
      | enSeatMoveCmd.EN_NULL == MotorCmd...
      | && (FALSE != UpForwardVolt...
      | || FALSE != DownBackwardVolt)]
  Normal -> Judge [order 2] : [/*输出命令向前/向上命令却有向后/向下电压 */
      | enSeatMoveCmd.EN_UP_FORWARD == MotorCmd...
      | &&  FALSE != DownBackwardVolt]
  Normal -> Judge [order 3] : [/*输出命令向后/向下命令却有向前/向上电压 */
      | enSeatMoveCmd.EN_DN_BACKWARD  == MotorCmd...
      | &&  FALSE != UpForwardVolt]
  Judge -> Normal [order 1] : [/*继电器粘连消失：
      |  1、没有控制开启命令，同时没有电压输出，认为继电器粘连消失
      |  2、控制开启命令，存在对应的电压输出，认为继电器粘连消失*/
      | (enSeatMoveCmd.EN_NULL == MotorCmd...
      | && FALSE == UpForwardVolt...
      | && FALSE == DownBackwardVolt) ...
      | || (enSeatMoveCmd.EN_UP_FORWARD == MotorCmd...
      | && TRUE == UpForwardVolt ...
      | && FALSE == DownBackwardVolt) ...
      | || (enSeatMoveCmd.EN_DN_BACKWARD == MotorCmd ...
      | && FALSE == UpForwardVolt ...
      | && TRUE == DownBackwardVolt) ]
  data: MotorCmd input; UpForwardVolt input; DownBackwardVolt input; MidRelayFault output uint8; CAL_MotorRelayErr_2s parameter; D_Relay_DownBackFault parameter; D_Relay_UpFrontFault parameter; FALSE parameter; TRUE parameter; MidRelayTimer output uint8

== stateflow chart APPL_PaFaultDetection/LogicCtrl/AdheAndEffec/SwitchErrorDetection ==
  state Ts = GetCurMsTs [function]
  state OutTs = TimeDiffTs(lastTs,Ts) [function]
  state OutTs = GetDefTime(DefTs,Ts) [function]
  state HeightSwitchErrorDeal [parallel] [commented out]
    state Valid [commented out]
      (default) -> (junction 631) [commented out]
      HeightSwitchErrorDeal.Valid -> (junction 631) [commented out]
      (junction 631) -> (junction 617) [commented out] : /*持续有效时间超过90s，则诊断为开关粘滞故障*/
          | [TimeDiffTs(HeightSwTimer,GetCurMsTs()) >= CAL_ManualSwValid_90s]
      (junction 631) -> (junction 658) [commented out] : {HeightSwCmd = MtrCtrlFault_DRHeightSwitch;
          | HeightSwUpAdhesionFault = FALSE;
          | HeightSwDownAdhesionFault = FALSE;}
      (junction 617) -> (junction 660) [commented out] : {HeightSwCmd = enSeatMoveCmd.EN_NULL;
          | HeightSwTimer = GetDefTime(CAL_ManualSwValid_90s,GetCurMsTs());
          | HeightSwAdhesionFault = TRUE;}
      (junction 660) -> (junction 618) [commented out] : [enSeatMoveCmd.EN_UP_FORWARD == MtrCtrlFault_DRHeightSwitch]
      (junction 660) -> (junction 619) [commented out] : {HeightSwDownAdhesionFault = TRUE;}
      (junction 618) -> (junction 642) [commented out] : {HeightSwUpAdhesionFault = TRUE;}
      (junction 619) -> (junction 658) [commented out]
      (junction 642) -> (junction 619) [commented out]
      (junction 658) -> (junction 643) [commented out]
    state Invalid [commented out]
      en:
      HeightSwTimer = GetCurMsTs();
      HeightSwAdhesionFault = FALSE;
      HeightSwCmd = enSeatMoveCmd.EN_NULL;
      HeightSwUpAdhesionFault = FALSE;
      HeightSwDownAdhesionFault = FALSE;
      du:
      HeightSwTimer = GetCurMsTs();
    (default) -> HeightSwitchErrorDeal.Invalid [commented out]
    HeightSwitchErrorDeal.Invalid -> HeightSwitchErrorDeal.Valid [commented out] : /*开关有效 */
        | [enSeatMoveCmd.EN_NULL != MtrCtrlFault_DRHeightSwitch]
    HeightSwitchErrorDeal.Valid -> HeightSwitchErrorDeal.Invalid [commented out] : /* 跳变 无效 */
        | [enSeatMoveCmd.EN_NULL == MtrCtrlFault_DRHeightSwitch ...
        | || hasChanged(MtrCtrlFault_DRHeightSwitch)]
  state LengthSwitchErrorDeal [parallel]
    settings: executionOrder=1
    state Valid
      (default) -> (junction 633)
      (junction 633) -> (junction 629) [order 1] : /*持续有效时间超过90s，则诊断为开关粘滞故障*/
          | [TimeDiffTs(LengthSwTimer,GetCurMsTs()) >= CAL_ManualSwValid_90s]
      LengthSwitchErrorDeal.Valid -> (junction 633) [order 1]
      (junction 629) -> (junction 632) : {LengthSwCmd = enSeatMoveCmd.EN_NULL;
          | LengthSwTimer = GetDefTime(CAL_ManualSwValid_90s,GetCurMsTs());
          | LengthSwAdhesionFault = TRUE;}
      (junction 633) -> (junction 639) [order 2] : {LengthSwCmd = MtrCtrlFault_DRLengthSwitch;
          | LengthSwUpAdhesionFault = FALSE;
          | LengthSwDownAdhesionFault = FALSE;}
      (junction 632) -> (junction 634) [order 1] : [enSeatMoveCmd.EN_UP_FORWARD == MtrCtrlFault_DRLengthSwitch]
      (junction 632) -> (junction 635) [order 2] : {LengthSwDownAdhesionFault = TRUE;}
      (junction 634) -> (junction 638) : {LengthSwUpAdhesionFault = TRUE;}
      (junction 638) -> (junction 635)
      (junction 635) -> (junction 639)
      (junction 639) -> (junction 644)
    state Invalid
      en:
      LengthSwTimer = GetCurMsTs();
      LengthSwAdhesionFault = FALSE;
      LengthSwCmd = enSeatMoveCmd.EN_NULL;
      LengthSwUpAdhesionFault = FALSE;
      LengthSwDownAdhesionFault = FALSE;
      du:
      LengthSwTimer = GetCurMsTs();
    (default) -> LengthSwitchErrorDeal.Invalid
    LengthSwitchErrorDeal.Invalid -> LengthSwitchErrorDeal.Valid : /*开关有效  */
        | [enSeatMoveCmd.EN_NULL != MtrCtrlFault_DRLengthSwitch]
    LengthSwitchErrorDeal.Valid -> LengthSwitchErrorDeal.Invalid [order 1] : /* 跳变 无效 */
        | [enSeatMoveCmd.EN_NULL == MtrCtrlFault_DRLengthSwitch ...
        | || hasChanged(MtrCtrlFault_DRLengthSwitch)]
  state BackSwitchErrorDeal [parallel]
    settings: executionOrder=2
    state Valid
      (default) -> (junction 666)
      BackSwitchErrorDeal.Valid -> (junction 666) [order 1]
      (junction 666) -> (junction 667) [order 1] : /*持续有效时间超过90s，则诊断为开关粘滞故障*/
          | [TimeDiffTs(BackSwTimer,GetCurMsTs()) >= CAL_ManualSwValid_90s]
      (junction 666) -> (junction 670) [order 2] : {BackSwCmd = MtrCtrlFault_DRBackSwitch;
          | BackSwUpAdhesionFault = FALSE;
          | BackSwDownAdhesionFault = FALSE;}
      (junction 667) -> (junction 668) : {BackSwCmd = enSeatMoveCmd.EN_NULL;
          | BackSwTimer = GetDefTime(CAL_ManualSwValid_90s,GetCurMsTs());
          | BackSwAdhesionFault = TRUE;}
      (junction 668) -> (junction 669) [order 1] : [enSeatMoveCmd.EN_UP_FORWARD == MtrCtrlFault_DRBackSwitch]
      (junction 668) -> (junction 671) [order 2] : {BackSwDownAdhesionFault = TRUE;}
      (junction 669) -> (junction 672) : {BackSwUpAdhesionFault = TRUE;}
      (junction 671) -> (junction 670)
      (junction 672) -> (junction 671)
      (junction 670) -> (junction 673)
    state Invalid
      en:
      BackSwTimer = GetCurMsTs();
      BackSwAdhesionFault = FALSE;
      BackSwCmd = enSeatMoveCmd.EN_NULL;
      BackSwUpAdhesionFault = FALSE;
      BackSwDownAdhesionFault = FALSE;
      du:
      BackSwTimer = GetCurMsTs();
    (default) -> BackSwitchErrorDeal.Invalid
    BackSwitchErrorDeal.Invalid -> BackSwitchErrorDeal.Valid : /*开关有效  */
        | [enSeatMoveCmd.EN_NULL != MtrCtrlFault_DRBackSwitch]
    BackSwitchErrorDeal.Valid -> BackSwitchErrorDeal.Invalid [order 1] : /* 跳变 无效 */
        | [enSeatMoveCmd.EN_NULL == MtrCtrlFault_DRBackSwitch ...
        | || hasChanged(MtrCtrlFault_DRBackSwitch)]
  state FrontSwitchErrorDeal [parallel] [commented out]
    state Valid [commented out]
      (default) -> (junction 690) [commented out]
      FrontSwitchErrorDeal.Valid -> (junction 690) [commented out]
      (junction 690) -> (junction 691) [commented out] : /*持续有效时间超过90s，则诊断为开关粘滞故障*/
          | [TimeDiffTs(FrontSwTimer,GetCurMsTs()) >= CAL_ManualSwValid_90s]
      (junction 690) -> (junction 694) [commented out] : {FrontSwCmd = MtrCtrlFault_DRFrontSwitch;
          | FrontSwUpAdhesionFault = FALSE;
          | FrontSwDownAdhesionFault = FALSE;}
      (junction 691) -> (junction 692) [commented out] : {FrontSwCmd = enSeatMoveCmd.EN_NULL;
          | FrontSwTimer = GetDefTime(CAL_ManualSwValid_90s,GetCurMsTs());
          | FrontSwAdhesionFault = TRUE;}
      (junction 692) -> (junction 693) [commented out] : [enSeatMoveCmd.EN_UP_FORWARD == MtrCtrlFault_DRFrontSwitch]
      (junction 692) -> (junction 695) [commented out] : {FrontSwDownAdhesionFault = TRUE;}
      (junction 693) -> (junction 696) [commented out] : {FrontSwUpAdhesionFault = TRUE;}
      (junction 695) -> (junction 694) [commented out]
      (junction 696) -> (junction 695) [commented out]
      (junction 694) -> (junction 697) [commented out]
    state Invalid [commented out]
      en:
      FrontSwTimer = GetCurMsTs();
      FrontSwAdhesionFault = FALSE;
      FrontSwCmd = enSeatMoveCmd.EN_NULL;
      FrontSwUpAdhesionFault = FALSE;
      FrontSwDownAdhesionFault = FALSE;
      du:
      FrontSwTimer = GetCurMsTs();
    (default) -> FrontSwitchErrorDeal.Invalid [commented out]
    FrontSwitchErrorDeal.Invalid -> FrontSwitchErrorDeal.Valid [commented out] : /*开关有效  */
        | [enSeatMoveCmd.EN_NULL != MtrCtrlFault_DRFrontSwitch]
    FrontSwitchErrorDeal.Valid -> FrontSwitchErrorDeal.Invalid [commented out] : /* 跳变 无效 */
        | [enSeatMoveCmd.EN_NULL == MtrCtrlFault_DRFrontSwitch ...
        | || hasChanged(MtrCtrlFault_DRFrontSwitch)]
  data: Ts function_output; lastTs function_input; Ts function_input; OutTs function_output; DefTs function_input; Ts function_input; OutTs function_output; MtrCtrlFault_DRHeightSwitch input; MtrCtrlFault_DRLengthSwitch input; MtrCtrlFault_DRBackSwitch input; MtrCtrlFault_DRFrontSwitch input; HeightSwAdhesionFault output uint8; LengthSwAdhesionFault output uint8; BackSwAdhesionFault output uint8; FrontSwAdhesionFault output uint8; HeightSwTimer local uint32; TRUE parameter; FALSE parameter; LengthSwTimer local uint32; BackSwTimer local uint32; FrontSwTimer local uint32; CAL_ManualSwValid_90s parameter; HeightSwCmd output Enum: enSeatMoveCmd; LengthSwCmd output Enum: enSeatMoveCmd; BackSwCmd output Enum: enSeatMoveCmd; FrontSwCmd output Enum: enSeatMoveCmd; LengthSwUpAdhesionFault output uint8; LengthSwDownAdhesionFault output uint8; BackSwUpAdhesionFault output uint8; BackSwDownAdhesionFault output uint8
